simulink model "Fahrstuhl"  (R2019a)
settings: Solver=FixedStepDiscrete  StartTime=0.0  StopTime=inf  FixedStep=1  RelTol=1e-3
settings Model: Creator=Naveen  LastModifiedBy=Naveen

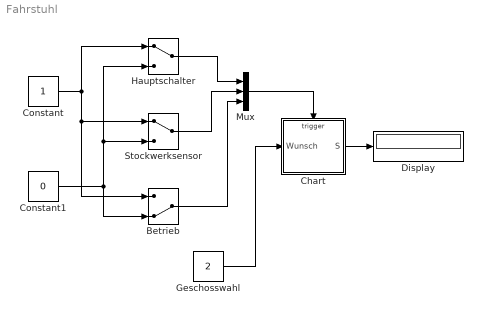
== system Fahrstuhl ==
  Betrieb : ManualSwitch  CurrentSetting=0
  Chart : Stateflow chart  BlockKeywords=__PRM__SERIALIZED__DATA__:Stateflow Chart,Stateflow Diagram  TreatAsAtomicUnit=on
  Constant : Constant
  Constant1 : Constant  Value=0
  Display : Display
  Geschosswahl : Constant  Value=2
  Hauptschalter : ManualSwitch
  Mux : Mux  Inputs=3
  Stockwerksensor : ManualSwitch
  wires:
  Hauptschalter/1 -> Mux/1
  Stockwerksensor/1 -> Mux/2
  Betrieb/1 -> Mux/3
  Mux/1 -> Chart/Trigger
  Chart/1(S) -> Display/1
  Geschosswahl/1 -> Chart/1(Wunsch)
  Constant1/1 -> Hauptschalter/2, Stockwerksensor/2, Betrieb/2
  Constant/1 -> Hauptschalter/1, Betrieb/1, Stockwerksensor/1

== stateflow chart Fahrstuhl/Chart ==
  settings: executeAtInitialization=1
  state Tuer [parallel]
    settings: executionOrder=1
    state Zu
      state Position
        (history)
        state StockZwei
          entry: S=2;
        state StockEins
          entry: S=1;
        state EU
          entry: S=0;
        state UG
          entry: S=-1;
        StockZwei -> StockEins : runter
        StockEins -> StockZwei [order 1] : hoch
        StockEins -> EU [order 2] : runter
        EU -> StockEins [order 1] : hoch
        (default) -> EU
        EU -> UG [order 2] : runter
        UG -> EU : hoch
    state Auf
    (default) -> Auf
    Auf -> Position : schliessen
    Position -> Auf : oeffnen
  state Fahrbetrieb [parallel]
    settings: executionOrder=2
    state Aus
    state Fahre_hoch
      on Stockwerksensor:hoch;
    state Bereitschaft
    state Fahre_runter
      on Stockwerksensor:runter;
    (default) -> Aus
    Aus -> Bereitschaft : Hauptschalter
    Bereitschaft -> Aus [order 1] : Hauptschalter
    (junction 38) -> Fahre_hoch [order 1] : [Z>S]
    Fahre_hoch -> (junction 42) : Stockwerksensor[Z-1==S]/hoch
    Bereitschaft -> (junction 38) [order 2] : Betrieb{Z=Wunsch}/schliessen
    Fahre_runter -> (junction 42) : Stockwerksensor[Z+1==S]/runter
    (junction 42) -> Bereitschaft : /oeffnen
    (junction 38) -> Fahre_runter [order 2] : [Z<S]
  data: Wunsch input double; S output double =0; Z local double
  events: Hauptschalter input EITHER_EDGE_EVENT; schliessen local FUNCTION_CALL_EVENT; oeffnen local FUNCTION_CALL_EVENT; hoch local FUNCTION_CALL_EVENT; runter local FUNCTION_CALL_EVENT; Stockwerksensor input EITHER_EDGE_EVENT; Betrieb input EITHER_EDGE_EVENT
